simulink model "pendulum_linearized"  (R2018b)
settings: Solver=VariableStepAuto  StartTime=0.0  StopTime=10.0  RelTol=1e-3
values from neighbouring files (symbols this model uses):
  A = [0 1 0 0;(g/L) 0 0 0; 0 0 0 1; 0 0 0 0]    [inverted_pendulum.m]    (also in inverted_pendulum_final.m)
  B = [0; -(1/L); 0; 1]    [inverted_pendulum.m]    (also in inverted_pendulum_final.m)
  C = [1 0 0 0; 0 0 1 0]    [inverted_pendulum.m]    (also in inverted_pendulum_final.m)
  D = [0; 0]    [inverted_pendulum.m]    (also in inverted_pendulum_final.m)
settings Model: Creator=ipebo  LastModifiedBy=ipebo

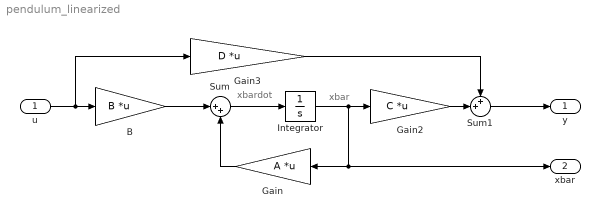
== system pendulum_linearized ==
  note: xbardot
  note: xbar
  u : Inport
  B : Gain  Gain=B  Multiplication=Matrix(K*u) (u vector)
  Gain : Gain  Gain=A  Multiplication=Matrix(K*u) (u vector)
  Gain2 : Gain  Gain=C  Multiplication=Matrix(K*u) (u vector)
  Gain3 : Gain  Gain=D  Multiplication=Matrix(K*u) (u vector)
  Integrator : Integrator
  Sum : Sum  Inputs=|++
  Sum1 : Sum  Inputs=++|
  y : Outport
  xbar : Outport  Port=2
  wires:
  Gain3/1 -> Sum1/1
  u/1 -> Gain3/1, B/1
  Gain/1 -> Sum/2
  Sum1/1 -> y/1
  Sum/1 -> Integrator/1
  Integrator/1 -> Gain/1, xbar/1, Gain2/1
  B/1 -> Sum/1
  Gain2/1 -> Sum1/2
